simulink model "sampleModel1569_2"  (R2023a)
settings: Solver=VariableStepAuto  StartTime=0.0  StopTime=10.0  RelTol=1e-3
libraries: hdlsllib x5, simulink x1
settings Model: Creator=user1  LastModifiedBy=user1

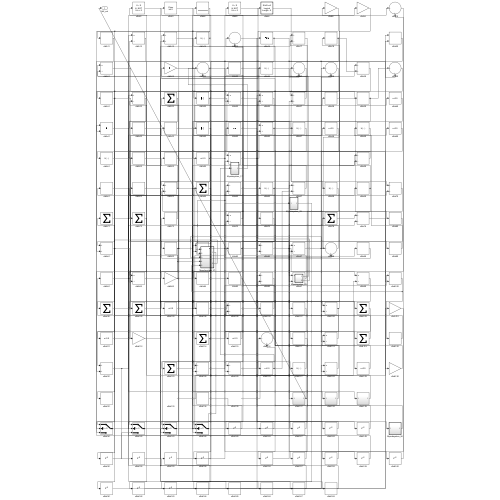
[thumbnail: Simulink's stored preview of the top-level diagram]
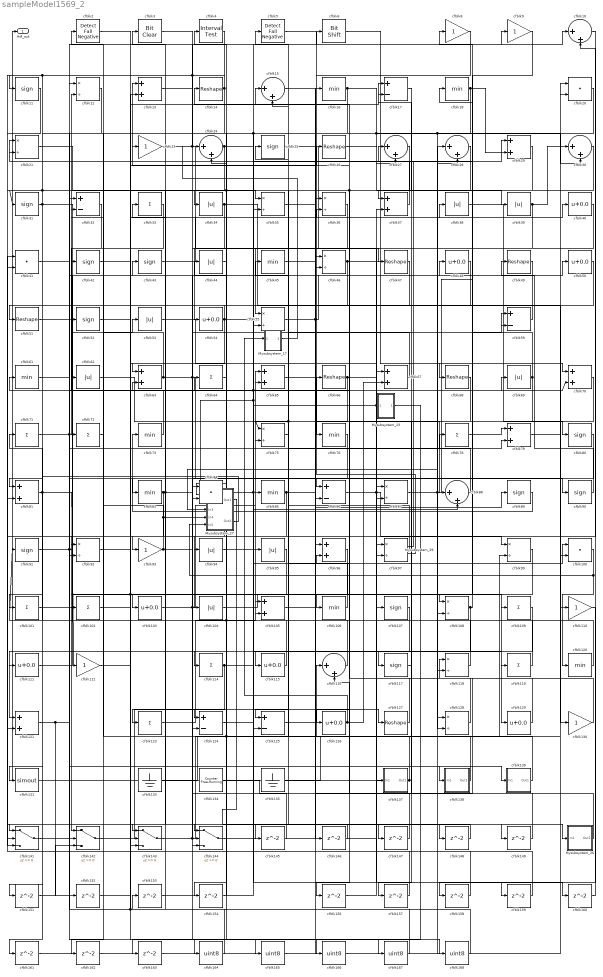
== system sampleModel1569_2 ==
  Mysubsystem_17 : Subsystem  TreatAsAtomicUnit=on  RTWFcnName=Mysubsystem_17
      settings: RTWFcnNameOpts=User specified  RTWFileNameOpts=Use function name
  Mysubsystem_23 : Subsystem  TreatAsAtomicUnit=on  RTWFcnName=Mysubsystem_23
      settings: RTWFcnNameOpts=User specified  RTWFileNameOpts=Use function name
  Mysubsystem_26 : Subsystem  TreatAsAtomicUnit=on  RTWFcnName=Mysubsystem_26
      settings: RTWFcnNameOpts=User specified  RTWFileNameOpts=Use function name
  Mysubsystem_27 : Subsystem  TreatAsAtomicUnit=on  RTWFcnName=Mysubsystem_27
      settings: RTWFcnNameOpts=User specified  RTWFileNameOpts=Use function name
  Mysubsystem_29 : Subsystem  TreatAsAtomicUnit=on  RTWFcnName=Mysubsystem_29
      settings: RTWFcnNameOpts=User specified  RTWFileNameOpts=Use function name
  cfblk{10,15,24,27..28,30,88,116} (8 alike) : Sum  Inputs=|++  OutDataTypeStr=uint8
  cfblk{20,41,84,100} (4 alike) : DotProduct  OutDataTypeStr=uint8
  cfblk{33,64,71..72,78,101..102,109,114,119,123} (11 alike) : Sum  Inputs=+  OutDataTypeStr=uint8
  cfblk{40,48,50,54,103,111,115,126,129} (9 alike) : Bias  Bias=0.0  SaturateOnIntegerOverflow=off
  cfblk{34,38..39,44,53,62,69,94..95,104} (10 alike) : Abs  OutDataTypeStr=uint8  SaturateOnIntegerOverflow=off
  cfblk{13,29,37,63,65,67,70,79,81,96,105,121} (12 alike) : Sum  OutDataTypeStr=uint8
  cfblk{16,18,45,61,73,76,83,85,106,120} (10 alike) : MinMax  OutDataTypeStr=uint8
  cfblk{11,25,31,42..43,52,80,89..91,107,117} (12 alike) : Signum
  cfblk{12,21,35..36,46,55,75,87,92,97,99,108,118,128} (14 alike) : Product  Inputs=*/  OutDataTypeStr=uint8  RndMeth=Zero  SaturateOnIntegerOverflow=on
  cfblk{8..9,23,93,110,112,130} (7 alike) : Gain  OutDataTypeStr=uint8
  cfblk{17,32,59,86,124..125} (6 alike) : Sum  Inputs=+-  OutDataTypeStr=uint8
  cfblk{14,26,47,49,51,66,68,127} (8 alike) : Reshape
  cfblk131 : ToWorkspace  VariableName=simout  SaveFormat=Timeseries  SampleTime=-1
  cfblk133 : Ground
  cfblk134 : hdlsllib/Sources/Counter Free-Running  NumBits=16  tsamp=-1
  cfblk135 : Ground
  cfblk137 : Subsystem
      settings: LibrarySourceBlock=|
      | hdlsllib/Ports &
      | Subsystems/Subsystem
  cfblk138 : Subsystem
      settings: LibrarySourceBlock=|
      | hdlsllib/Ports &
      | Subsystems/Subsystem
  cfblk139 : Subsystem
      settings: LibrarySourceBlock=|
      | hdlsllib/Ports &
      | Subsystems/Subsystem
  cfblk{141..144} (4 alike) : Switch  OutDataTypeStr=uint8  SaturateOnIntegerOverflow=off  InputSameDT=off
  cfblk{145..149,151..154,156..163} (17 alike) : Delay  SampleTime=1
  cfblk{164..168} (5 alike) : DataTypeConversion  OutDataTypeStr=uint8  SaturateOnIntegerOverflow=off  RndMeth=Floor
  cfblk2 : hdlsllib/Logic and Bit Operations/Detect Fall Negative  vinit=0  OutDataTypeStr=uint8
  cfblk3 : simulink/Logic and Bit Operations/Bit Clear  iBit=0
      settings: LibrarySourceBlock=|
      | hdlsllib/Logic and Bit
      | Operations/Bit Clear
  cfblk4 : hdlsllib/Logic and Bit Operations/Interval Test  IntervalClosedRight=on  uplimit=0.5  IntervalClosedLeft=on  lowlimit=-0.5  OutDataTypeStr=uint8
  cfblk5 : hdlsllib/Logic and Bit Operations/Detect Fall Negative  vinit=0  OutDataTypeStr=uint8
  cfblk6 : hdlsllib/Logic and Bit Operations/Bit Shift  mode=Shift Left Logical  N=0
  Hdl_out : Outport  OutDataTypeStr=uint8
  wires:
  cfblk91/1 -> cfblk48/1, cfblk9/1
  cfblk87/1 -> Mysubsystem_27/3(In3), cfblk21/1
  cfblk5/1 -> cfblk76/1
  cfblk29/1 -> cfblk75/1, cfblk145/1
  cfblk118/1 -> cfblk91/1, cfblk44/1
  cfblk107/1 -> cfblk117/1
  cfblk37/1 -> cfblk13/1
  cfblk138/1(Out1) -> cfblk116/1
  cfblk104/1 -> cfblk129/1
  cfblk46/1 -> cfblk70/1, cfblk123/1
  cfblk10/1 -> cfblk93/1
  cfblk134/1 -> cfblk118/1
  cfblk89/1 -> cfblk73/1
  cfblk54/1 -> Mysubsystem_27/2(In2), cfblk160/1, cfblk6/1, cfblk51/1, cfblk143/3
  cfblk99/1 -> cfblk106/1
  cfblk119/1 -> cfblk65/1
  cfblk121/1 -> cfblk75/2, cfblk152/1
  cfblk108/1 -> cfblk8/1, cfblk125/2
  cfblk63/1 -> cfblk137/1(In1), cfblk127/1, cfblk2/1
  cfblk84/1 -> Mysubsystem_23/1(In1), cfblk119/1, cfblk142/1
  cfblk8/1 -> cfblk46/1
  cfblk127/1 -> cfblk14/1
  cfblk36/1 -> cfblk55/1
  cfblk141/1 -> cfblk43/1
  cfblk68/1 -> cfblk86/1
  cfblk39/1 -> cfblk30/1, cfblk114/1
  cfblk66/1 -> cfblk86/2, cfblk59/1
  cfblk111/1 -> cfblk64/1
  cfblk50/1 -> cfblk118/2
  cfblk100/1 -> Mysubsystem_27/5(In5), cfblk120/1
  cfblk47/1 -> cfblk115/1
  cfblk125/1 -> cfblk46/2
  cfblk123/1 -> cfblk105/1
  cfblk6/1 -> cfblk68/1
  cfblk124/1 -> cfblk95/1
  cfblk103/1 -> cfblk85/1, cfblk78/1
  cfblk93/1 -> cfblk21/2, Mysubsystem_27/4(In4), cfblk59/2
  cfblk38/1 -> cfblk80/1
  cfblk97/1 -> cfblk15/1
  cfblk51/1 -> cfblk109/1
  cfblk78/1 -> cfblk79/1
  cfblk21/1 -> cfblk35/1
  cfblk23/1 -> cfblk47/1, cfblk10/1
  cfblk96/1 -> cfblk103/1
  cfblk94/1 -> cfblk29/1, cfblk70/2
  cfblk102/1 -> cfblk17/1
  cfblk31/1 -> cfblk90/1, cfblk131/1
  cfblk83/1 -> cfblk50/1, cfblk33/1, cfblk121/2
  cfblk88/1 -> cfblk25/1
  cfblk25/1 -> cfblk97/1
  cfblk112/1 -> cfblk40/1
  cfblk142/1 -> cfblk124/1
  cfblk101/1 -> cfblk53/1
  cfblk143/1 -> cfblk110/1, cfblk79/2
  cfblk133/1 -> cfblk67/1
  cfblk2/1 -> cfblk108/2, cfblk165/1
  cfblk4/1 -> cfblk141/1, cfblk141/3, cfblk124/2
  cfblk109/1 -> cfblk121/1
  cfblk67/1 -> cfblk5/1
  cfblk137/1(Out1) -> cfblk4/1, cfblk32/2, Hdl_out/1
  cfblk81/1 -> cfblk112/1, cfblk161/1
  cfblk73/1 -> cfblk12/2
  cfblk14/1 -> cfblk11/1, cfblk92/2
  cfblk33/1 -> cfblk72/1
  cfblk32/1 -> cfblk42/1
  cfblk30/1 -> cfblk111/1, cfblk126/1
  cfblk52/1 -> cfblk26/1
  cfblk13/1 -> cfblk138/1(In1)
  cfblk86/1 -> cfblk99/1, cfblk159/1
  cfblk34/1 -> cfblk130/1, cfblk144/3
  cfblk28/1 -> cfblk34/1
  cfblk71/1 -> cfblk69/1, cfblk139/1(In1)
  cfblk26/1 -> cfblk27/2
  cfblk48/1 -> cfblk81/1
  cfblk120/1 -> cfblk105/2
  cfblk53/1 -> cfblk107/1
  cfblk11/1 -> cfblk81/2
  cfblk80/1 -> cfblk125/1
  cfblk126/1 -> Mysubsystem_17/1(In1), cfblk67/2
  cfblk135/1 -> cfblk99/2
  cfblk42/1 -> cfblk84/2
  cfblk106/1 -> cfblk65/2
  cfblk139/1(Out1) -> cfblk15/2
  cfblk75/1 -> cfblk45/1
  cfblk128/1 -> cfblk23/1
  cfblk44/1 -> cfblk144/1
  cfblk62/1 -> cfblk88/1
  cfblk41/1 -> cfblk83/1
  cfblk129/1 -> cfblk61/1
  cfblk76/1 -> cfblk144/2
  cfblk114/1 -> cfblk100/1, cfblk143/1
  cfblk85/1 -> cfblk104/1, cfblk38/1
  cfblk144/1 -> cfblk87/1
  cfblk17/1 -> cfblk37/1
  cfblk105/1 -> cfblk89/1
  cfblk130/1 -> cfblk96/2
  cfblk79/1 -> cfblk100/2
  cfblk18/1 -> cfblk94/1, cfblk128/2, cfblk29/2
  cfblk24/1 -> cfblk63/1, cfblk88/2
  cfblk95/1 -> cfblk102/1
  cfblk16/1 -> cfblk92/1, cfblk35/2, cfblk30/2, cfblk39/1
  cfblk59/1 -> cfblk52/1
  cfblk115/1 -> cfblk62/1
  cfblk69/1 -> cfblk18/1, cfblk97/2
  cfblk65/1 -> cfblk16/1
  cfblk40/1 -> cfblk54/1
  cfblk116/1 -> cfblk71/1
  cfblk90/1 -> cfblk49/1
  cfblk9/1 -> cfblk108/1
  cfblk55/1 -> cfblk28/2, cfblk87/2
  cfblk12/1 -> cfblk31/1, cfblk101/1
  cfblk3/1 -> cfblk168/1
  cfblk27/1 -> Mysubsystem_27/1(In1), cfblk41/2
  cfblk43/1 -> cfblk36/2
  cfblk145/1 -> cfblk84/1
  cfblk45/1 -> cfblk146/1
  cfblk146/1 -> cfblk141/2
  cfblk70/1 -> cfblk147/1
  cfblk147/1 -> cfblk116/2
  cfblk15/1 -> cfblk148/1
  cfblk148/1 -> cfblk142/2
  cfblk35/1 -> cfblk149/1
  cfblk149/1 -> cfblk96/1
  cfblk151/1 -> cfblk142/3
  cfblk152/1 -> cfblk13/2
  cfblk153/1 -> cfblk55/2
  cfblk64/1 -> cfblk154/1
  cfblk154/1 -> cfblk24/2
  cfblk49/1 -> cfblk156/1
  cfblk156/1 -> cfblk37/2
  cfblk117/1 -> cfblk157/1
  cfblk157/1 -> cfblk12/1
  cfblk110/1 -> cfblk158/1
  cfblk158/1 -> cfblk41/1
  cfblk159/1 -> cfblk63/2
  cfblk160/1 -> cfblk10/2
  cfblk161/1 -> cfblk128/1
  cfblk72/1 -> cfblk162/1
  cfblk162/1 -> cfblk36/1
  cfblk163/1 -> cfblk28/1
  cfblk20/1 -> cfblk164/1
  cfblk164/1 -> cfblk153/1
  cfblk165/1 -> cfblk20/1
  cfblk92/1 -> cfblk166/1
  cfblk166/1 -> cfblk20/2
  cfblk61/1 -> cfblk167/1
  cfblk167/1 -> cfblk3/1
  cfblk168/1 -> cfblk143/2, cfblk32/1
  Mysubsystem_17/1(Out1) -> cfblk24/1
  Mysubsystem_23/1(Out1) -> cfblk163/1
  Mysubsystem_26/1(Out1) -> cfblk17/2
  Mysubsystem_27/1(Out1) -> Mysubsystem_26/1(In1)
  Mysubsystem_27/2(Out2) -> cfblk151/1
  Mysubsystem_29/1(Out1) -> cfblk27/1
  Mysubsystem_29/2(Out2) -> cfblk66/1

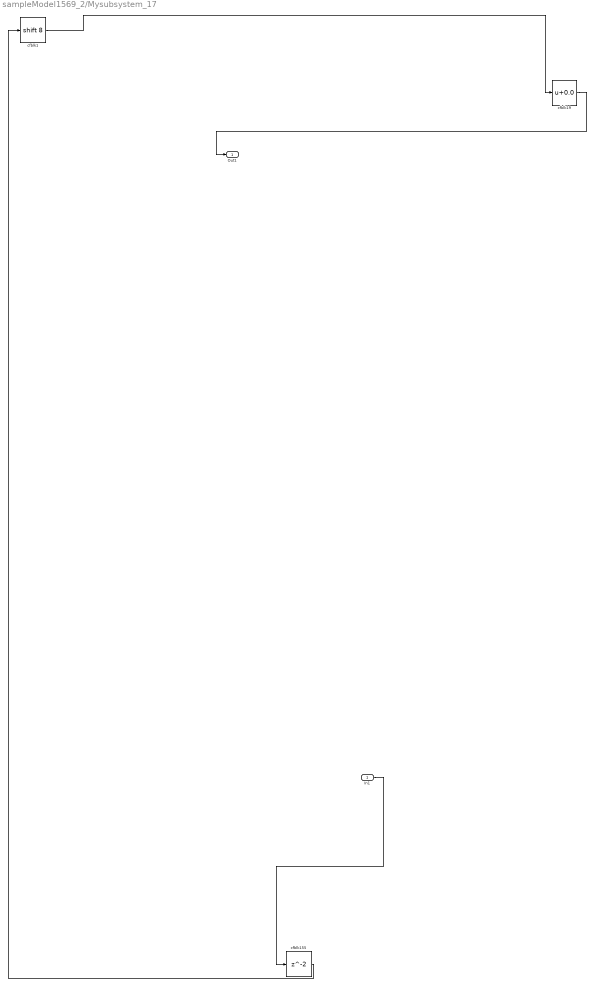
== system sampleModel1569_2/Mysubsystem_17 ==
  In1 : Inport
  cfblk1 : ArithShift  BitShiftNumber=8
  cfblk155 : Delay  SampleTime=1
  cfblk19 : Bias  Bias=0.0  SaturateOnIntegerOverflow=off
  Out1 : Outport
  wires:
  cfblk155/1 -> cfblk1/1
  cfblk1/1 -> cfblk19/1
  cfblk19/1 -> Out1/1
  In1/1 -> cfblk155/1

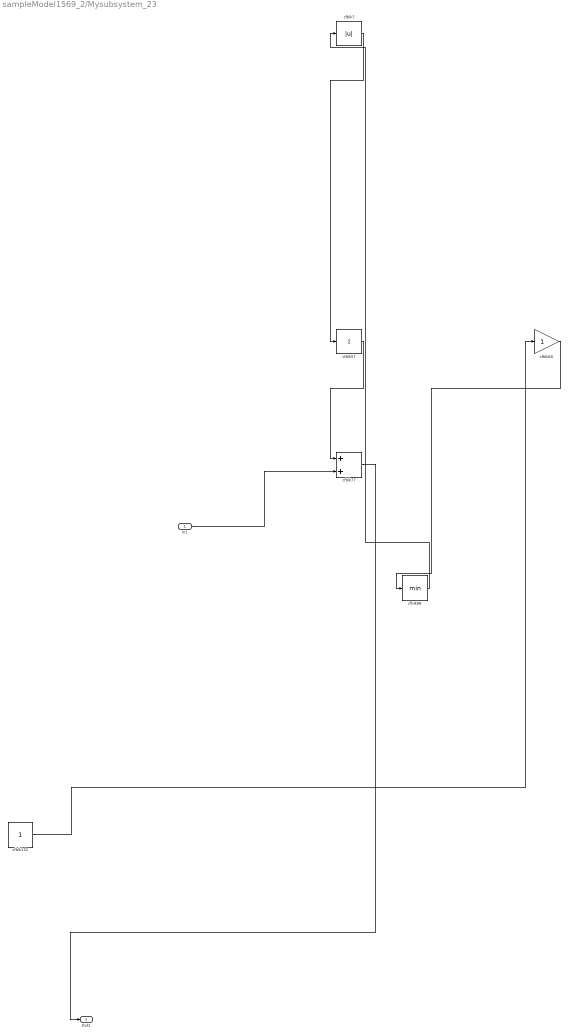
== system sampleModel1569_2/Mysubsystem_23 ==
  In1 : Inport
  cfblk132 : Constant  SampleTime=-1
  cfblk57 : Sum  Inputs=+
  cfblk60 : Gain
  cfblk7 : Abs  SaturateOnIntegerOverflow=off
  cfblk77 : Sum
  cfblk98 : MinMax
  Out1 : Outport
  wires:
  cfblk60/1 -> cfblk98/1
  cfblk132/1 -> cfblk60/1
  In1/1 -> cfblk77/2
  cfblk57/1 -> cfblk77/1
  cfblk7/1 -> cfblk57/1
  cfblk98/1 -> cfblk7/1
  cfblk77/1 -> Out1/1

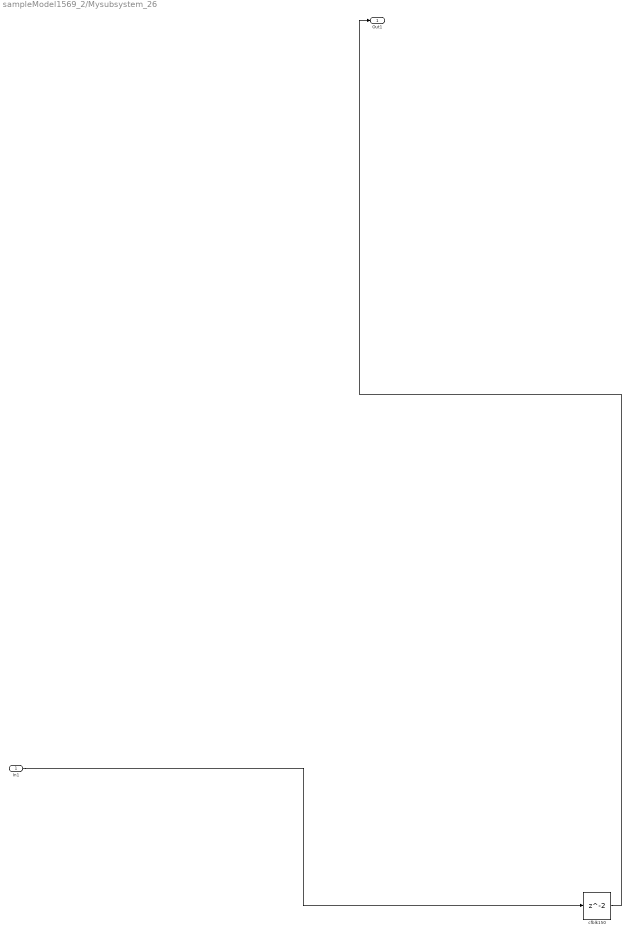
== system sampleModel1569_2/Mysubsystem_26 ==
  In1 : Inport
  cfblk150 : Delay  SampleTime=1
  Out1 : Outport
  wires:
  In1/1 -> cfblk150/1
  cfblk150/1 -> Out1/1

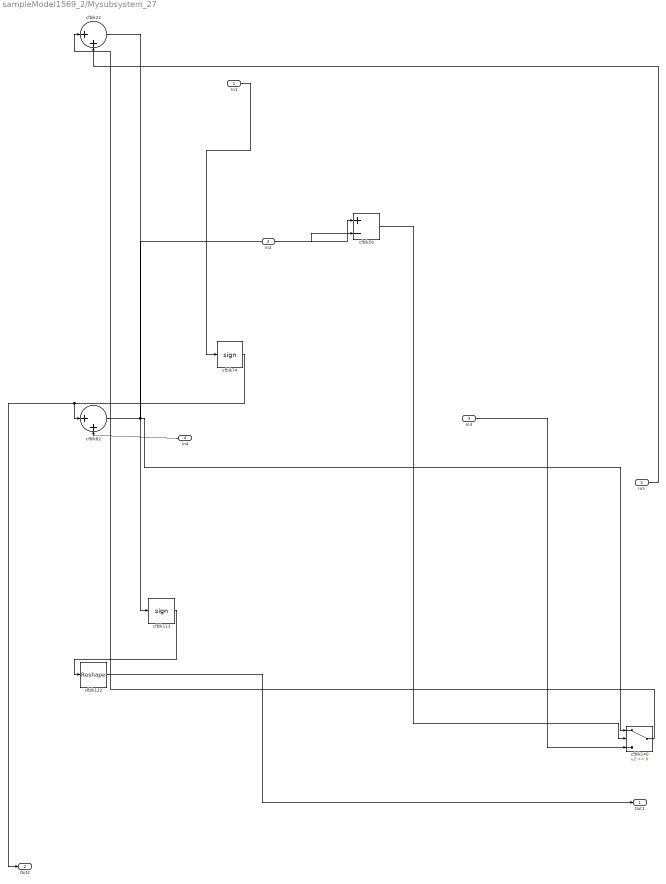
== system sampleModel1569_2/Mysubsystem_27 ==
  In1 : Inport
  In2 : Inport  Port=2
  In3 : Inport  Port=3
  In4 : Inport  Port=4
  In5 : Inport  Port=5
  cfblk113 : Signum
  cfblk122 : Reshape
  cfblk140 : Switch  SaturateOnIntegerOverflow=off  InputSameDT=off
  cfblk22 : Sum  Inputs=|++
  cfblk56 : Sum  Inputs=+-
  cfblk74 : Signum
  cfblk82 : Sum  Inputs=|++
  Out1 : Outport
  Out2 : Outport  Port=2
  wires:
  cfblk22/1 -> cfblk113/1
  cfblk74/1 -> Out2/1, cfblk82/1
  In5/1 -> cfblk22/2
  cfblk82/1 -> cfblk140/1, cfblk56/1
  cfblk140/1 -> cfblk22/1
  In3/1 -> cfblk140/3
  cfblk56/1 -> cfblk140/2
  cfblk113/1 -> cfblk122/1
  In1/1 -> cfblk74/1
  cfblk122/1 -> Out1/1
  In4/1 -> cfblk82/2
  In2/1 -> cfblk56/2

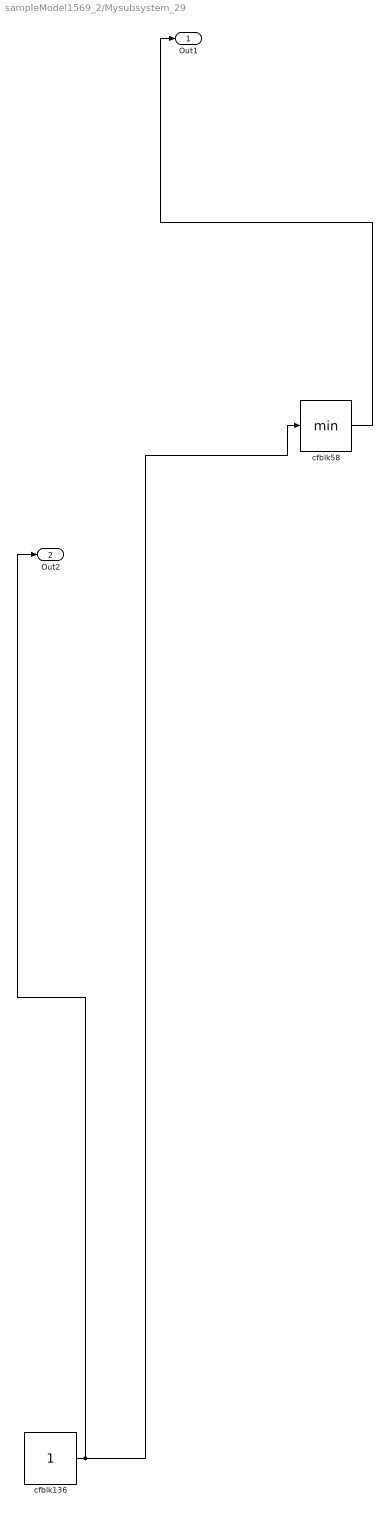
== system sampleModel1569_2/Mysubsystem_29 ==
  cfblk136 : Constant  SampleTime=-1
  cfblk58 : MinMax
  Out1 : Outport
  Out2 : Outport  Port=2
  wires:
  cfblk136/1 -> Out2/1, cfblk58/1
  cfblk58/1 -> Out1/1

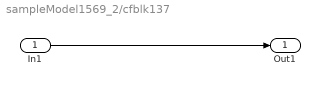
== system sampleModel1569_2/cfblk137 ==
  In1 : Inport
  Out1 : Outport
  wires:
  In1/1 -> Out1/1

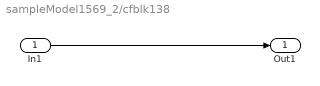
== system sampleModel1569_2/cfblk138 ==
  In1 : Inport
  Out1 : Outport
  wires:
  In1/1 -> Out1/1

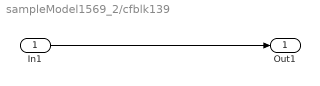
== system sampleModel1569_2/cfblk139 ==
  In1 : Inport
  Out1 : Outport
  wires:
  In1/1 -> Out1/1
